simulink model "Lab3_HallLog_hw"  (R2025b)
settings: Solver=FixedStepDiscrete  StartTime=0.0  StopTime=inf  FixedStep=50e-6  RelTol=1e-3  EnableMultiTasking=on
undefined symbols (not defined in the file or in its folder): A0, A4, ADC, B0, C10, C11, C12, C13, C14, C15, C2, C3, C4, C5, D0, D1, D10, D12, D13, D14, D2, D3, D5, D6, D9, DiscIntNeverNeededParam, Max, MaxPer, ms, NumBits1, NumBits2, P1, P17, P20, P35, P36, P37, P38, P43, P44, P45, P46, P47, P48, P49, P50, P51, P52, P54, P55, P58, P59, P61, P62, P63, Pin, PWM1_Trg1, Resol, s, us
libraries: simulink x29, MCHP_Blockset x18
(part 2 of 4)

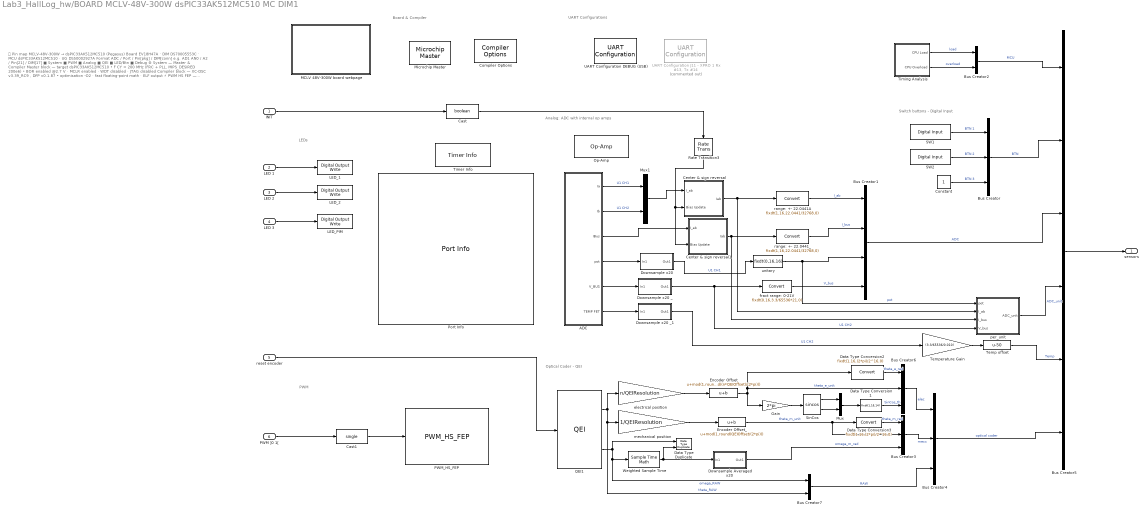
== system Lab3_HallLog_hw/BOARD MCLV-48V-300W dsPIC33AK512MC510 MC DIM1 ==
  note: Switch buttons - Digital Input
  note: LEDs
  note: UART Configurations
  note: PWM
  note: Optical Coder - QEI
  note: Analog: ADC with internal op amps
  note: Board & Compiler
  note: 🔌 Pin map MCLV-48V-300W → dsPIC33AK512MC510 (Pegasus)
      | Board EV18H47A · DIM DS70005553C · MCU dsPIC33AK512MC510 · UG DS50002927A
      | Format ADC / Port / Pin[pkg] / DIM[conn] e.g. AD1 AN0 / A2 / Pin[21] / DIM[17]
      | ■ System ■ PWM ■ Analog ■ QEI ■ LED/Btn ■ Debug
      | ⚙ System — Master & Compiler
      | Master block — target dsPIC33AK512MC510
      | • F CY = 200 MHz (FRC + PLL, MIPS_DESIRED 200e6)
      | • BOR enabled @2.7 V · MCLR enabled · WDT disabled · JTAG disabled
      | Compiler block — XC-DSC v3.39_RC9 , DFP v0.1.87
      | • optimisation -O2 · fast floating-point math · ELF output
      | ⚡ PWM HS FEP — 3-phase motor drive
      | PWM_HS_FEP — center-aligned, complementary (H/L pairs):
      | • period 50 µs = 20 kHz · dead-time 2 µs · resolution 0.275 µs
      | • PG1 triggers ADC (conversion synced to PWM) · channels 1-3 used
      | RD2 / Pin[82] / DIM[ 1] M1_PWM_AH RD3 / Pin[83] / DIM[ 3] M1_PWM_AL
      | RD0 / Pin[78] / DIM[ 5] M1_PWM_BH RD1 / Pin[79] / DIM[ 7] M1_PWM_BL
      | RC3 / Pin[66] / DIM[ 2] M1_PWM_CH RC4 / Pin[67] / DIM[ 4] M1_PWM_CL
      | 🌙 Analog — current & voltage sense
      | Phase & bus current — internal Op-Amp path (on-chip OA1/OA2/OA3 of the Pegasus DIM):
      | • R sh = 0.003 Ω × A v,DIM = 25 ⇒ 75 mV/A, biased at 1.65 V (V ref = Avdd/2)
      | • full scale = ±22.0441 A (firmware 22.0441/2^15 ) (DIM DS70005553C )
      | • External Op-Amp alt. : baseboard shunt 0.01 Ω + baseboard amp; jumpers DS50002927A Table 3-2
      | DC-bus voltage — resistor divider ( DS50002927A §3.2.5, Fig. 3-5) :
      | • R87/(R69+R77+R87) = 3.3/(34+34+3.3) = 1/21.6 ⇒ V bus,fs ≈ 69–71 V (firmware 3.3/2^16×21 )
      | AD1 AN0 / A2 / Pin[21] / DIM[17] M1_IA (OA1OUT)
      | AD2 AN0 / B0 / Pin[31] / DIM[25] M1_IB (OA2OUT)
      | AD3 AN0 / A5 / Pin[24] / DIM[33] M1_IBUS (OA3OUT)
      | A4 / Pin[23] OA1 IN+ A3 / Pin[22] OA1 IN-
      | B2 / Pin[33] OA2 IN+ B1 / Pin[32] OA2 IN-
      | B5 / Pin[26] OA3 IN+ A6 / Pin[25] OA3 IN-
      | ⚙ QEI · 💡 Digital I/O (LEDs & buttons)
      | LEDs = Digital Outputs · SW1/SW2 = Digital Inputs · QEI = quadrature encoder A/B.
      | RD14 / Pin[96] / DIM[42] M1_QEI_A RE2 / Pin[10] / DIM[30] M1_LED1 (DOut)
      | RD13 / Pin[95] / DIM[44] M1_QEI_B RE3 / Pin[ 6] / DIM[32] M1_LED2 (DOut)
      | RF1 / Pin[38] LED_DIM (DOut)
      | RA12 / Pin[ 3] / DIM[34] SW1 (M1_BUTTON1) (DIn)
      | RE1 / Pin[ 2] / DIM[36] SW2 (M1_BUTTON2) (DIn)
      | 🖥 Debug UART / programming
      | UART1 (DEBUG / USB) — 460800 baud , 8-N-1, Tx via DMA circular buffer.
      | Reaches the PC over the on-board USB-UART bridge → USB CDC virtual COM port
      | ( DS50002927A §2.2.3, J6) .
      | RC15 / Pin[75] / DIM[52] DEBUG_TX (U1TX)
      | RC14 / Pin[74] / DIM[54] DEBUG_RX (U1RX)
      | 🔗 Product page · Board User's Guide · DIM info sheet
  INIT : Inport
  LED 1 : Inport  Port=2
  LED 2 : Inport  Port=3
  LED 3 : Inport  Port=4
  reset encoder : Inport  Port=5
  PWM ]0 1[ : Inport  Port=6  Unit=1
  ADC : Subsystem
  Bus Creator{,3..4,6} (4 alike) : BusCreator  Inputs=3
  Bus Creator1 : BusCreator  Inputs=4
  Bus Creator2 : BusCreator  Inputs=2
  Bus Creator5 : BusCreator  Inputs=6
  Bus Creator7 : BusCreator  Inputs=2
  Cast : DataTypeConversion  OutDataTypeStr=boolean  SaturateOnIntegerOverflow=off  RndMeth=Floor
  Cast1 : DataTypeConversion  OutDataTypeStr=single  SaturateOnIntegerOverflow=off  RndMeth=Floor
  Center & sign reversal : Subsystem
  Center & sign reversal1 : Subsystem
  Compiler Options : MCHP_Blockset/System Configuration/Compiler Options  Priority=1  LATEST_CMPLR=on  COMP_LIST_TXT=XC-DSC - v4.00  DFP_LIST_TXT=v 1.4.172  CMSIS_DSP_TXT=Dynamic Options  USE_64BIT_DOUBLE=off  MCHP_MULTITHREAD_COMPILATION=on  UseCustom_LinkerScript=off  MCHP_MASTERLINK=Lab3_HallLog_hw_solution/BOARD MCLV-48V-300W dsPIC33AK512MC510 MC DIM1/Microchip Master  OPTIMIZATION_LEVEL=2  MPLAB_LINKLIB=default  MPLAB_LINKLIB1=fast floating-point math  CodeReplacement_TXT=None  OPTIMIZATION_FLTO=off  OPTIMIZATION_REORDER=off  OPTIMIZATION_ASM_REORDER=on  UNROLL_LOOPS=off  PROCEDURAL_ABSTRACTION=off  CONSERVE_STACK=off  GC_SECTIONS=None  MCODE=is more than 32768  MCONST=in data memory  MDATA=Can use all available memory  MSCALAR=Can use all available memory  MLARGEARRAY=off  MAGGREGATE=off  HEAP_SIZE=1024  OMF=elf  DEBUG_INFO=on  MCHP_STACK_USAGE=off  GCC_STACK_USAGE=off  ProduceHexOutput=off  AssemblyListing=off  SaveTemps=off  NO_EDS_WARN=on  PRINT_STATISTICS=off
      settings: SourceProductName=MPLAB Device Blocks for Simulink
  Constant : Constant  OutDataTypeStr=boolean  SampleTime=-1
  Data Type Duplicate : DataTypeDuplicate
  Data Type Conversion1 : DataTypeConversion  OutDataTypeStr=fixdt(1,16,14)  RndMeth=Floor
  Data Type Conversion2 : DataTypeConversion  OutDataTypeStr=fixdt(1,16,(2*pi)/2^16,0)  ConvertRealWorld=Stored Integer (SI)  SaturateOnIntegerOverflow=off  RndMeth=Floor
  Data Type Conversion3 : DataTypeConversion  OutDataTypeStr=fixdt(1,16,(2*pi)/2^16,0)  ConvertRealWorld=Stored Integer (SI)  SaturateOnIntegerOverflow=off  RndMeth=Floor
  Downsample Averaged x20 : Subsystem  mask{DownSample=10}
      mask prompts: DownSample "DownSample Factor"
  Downsample x20 : Subsystem  mask{DownSample=20}
      mask prompts: DownSample "DownSample Factor"
  Downsample x20 _ : Subsystem  mask{DownSample=20}
      mask prompts: DownSample "DownSample Factor"
  Downsample x20 _1 : Subsystem  mask{DownSample=20}
      mask prompts: DownSample "DownSample Factor"
  Encoder Offset : Bias  Bias=mod(1,round((n*QEIOffset)/(2*pi)))  SaturateOnIntegerOverflow=off
  Encoder Offset_ : Bias  Bias=mod(1,round(QEIOffset/(2*pi)))  SaturateOnIntegerOverflow=off
  Gain : Gain  Gain=2*pi  ParamDataTypeStr=single  OutDataTypeStr=single
  LED_1 : MCHP_Blockset/Digital IO/Digital Output Write  PORT_TXT="E   [ 0 : 4 ]"  PIN=2  INIT_VALUE=-1  PACK=off  OUTPUT_PIN_MODE=Push-Pull (default)  SIMULTANEOUS=off  ORDERING=None  SampleTime=-1  MCHP_PORT={Digital Out}{DOU}1:1:E2;  MCHP_MASTERLINK=Lab3_HallLog_hw_solution/BOARD MCLV-48V-300W dsPIC33AK512MC510 MC DIM1/Microchip Master
      settings: SourceProductName=MPLAB Device Blocks for Simulink
  LED_2 : MCHP_Blockset/Digital IO/Digital Output Write  PORT_TXT="E   [ 0 : 4 ]"  PIN=3  INIT_VALUE=-1  PACK=off  OUTPUT_PIN_MODE=Push-Pull (default)  SIMULTANEOUS=off  ORDERING=None  SampleTime=-1  MCHP_PORT={Digital Out}{DOU}1:1:E3;  MCHP_MASTERLINK=Lab3_HallLog_hw_solution/BOARD MCLV-48V-300W dsPIC33AK512MC510 MC DIM1/Microchip Master
      settings: SourceProductName=MPLAB Device Blocks for Simulink
  LED_PIM : MCHP_Blockset/Digital IO/Digital Output Write  PORT_TXT="F   [ 0 : 3 ]"  PIN=1  INIT_VALUE=-1  PACK=off  OUTPUT_PIN_MODE=Push-Pull (default)  SIMULTANEOUS=off  ORDERING=None  SampleTime=-1  MCHP_PORT={Digital Out}{DOU}1:1:F1;  MCHP_MASTERLINK=Lab3_HallLog_hw_solution/BOARD MCLV-48V-300W dsPIC33AK512MC510 MC DIM1/Microchip Master
      settings: SourceProductName=MPLAB Device Blocks for Simulink
  MCLV 48V-300W board webpage : Subsystem
      settings: OpenFcn=|
      | web('https://www.microchip.com/en-us/development-tool/EV62P66A','-browser'); % dsPIC33CK256MP508 DIM
      | pause(1);
      | web('https://www.microchip.com/en-us/development-tool/EV18H47A','-browser'); % LVMC 300W
      mask Display: image('MCHP_i_Board_MCLV_300W48V_reduced.jpg');
  Microchip Master : MCHP_Blockset/System Configuration/Microchip Master  Priority=1  PICREF=33AK512MC510  TIMESTEP_REF=PWM1_Trg1 + ADC  BUSYFLAG_TXT=None  PWRTEN=Not used  BOREN=Enabled  BODENV=2.7V  BORV=Not used  FPWRT=64ms  DSBOREN=Enable ZPBOR during Deep Sleep Mode  DSLPBOR=Not used  MCLRE=Enabled  SMCLR=MCLR pin generates a normal system Reset  PMDL1WAY=Allow only one reconfiguration  RSTPRI=Device will obtain reset instruction from Primary flash  TEMP=Not used  SOSCSRC=Not used  SOSCSEL=Not used  IOL1WAY=Allow only one reconfiguration  ALTVREF=Not used  DISUVREG=Not used  DSSWEN=Not used  LPCFG=Not used  RTCBAT=Not used  VBTBOR=Not used  WUTSEL=Not used  POWERSAVE=off  FNOSC=Internal Fast RC (FRC)  FPR=ECIO w/ PLL 16x  FOSFPR=Internal Fast RC (No change to Primary Osc Mode bits)  FOS=Primary Oscillator  FRANGE=High Range  OSCILLATOR_SELECT=External Clock  OSCILLATOR_SELECT_spd=External Clock  QUARTZ=8e6  QUARTZ_spd=8e6  FRC_TUNE_Range12_Step0P375=0.000 %  FRC_TUNE_Range12_Step0P375_CUSTOM=0  FRC_TUNE_Range1P5_Step0P047=0.000 %  FRC_TUNE_Range1P5_Step0P047_CUSTOM=0  BFRC_TUNE_Range1P5_Step0P047=0.000 %  BFRC_TUNE_Range1P5_Step0P047_CUSTOM=0  POSCGAIN=2x gain setting  POSCBOOST=Boost the kick start of the oscillator  SOSCGAIN=2x gain setting  SOSCBOOST=Boost the kick start of the oscillator  ACTIV_PLL=on  ACTIV_PLL_spd=on  MIPS_DESIRED=200e6  MIPS_DESIRED_spd=200e6  CPUDIV=Divide by 1  FPLLMUL=Not used  FPLLIDIV=8x Divider  POSCFREQ=Not used  POSCMD=Primary Oscillator Disabled  POSCMOD=Primary osc disabled  MIPS=200 * 1e6  ACLKCON=Optimized for PWM resolution & ADC conversion speed  ACLKCON_spd=Optimized for PWM resolution & ADC conversion speed  FPLLODIV=32x Divider  PLLKEN=Clock switch to PLL source will wait until the PLL lock signal is valid  FCKSM=Both Clock switching and Fail-safe Clock Monitor are disabled  FCKSMEN=Sw Disabled; Mon Disabled  IESO=Start up with FRC; then switch  DSWDTPS=1:2^36  FWDTEN=Disable  FWDTWINSZ=Window size is 25%  FWPSA=1:512  FWPSA0=1:128  FWPSB=1:16  WDT=Disable  WDTPOST=1:32768  WDTPRE=1:128  WDTPS=1:1048576  WINDIS=Watchdog Timer operates in Non-Window mode  WWDTEN=Non-Window mode  DSWDTEN=Enable DSWDT during Deep Sleep Mode  DSWDTOSC=Select LPRC as DSWDT Reference clock  FWDT_RCLKSEL=WDT Run Mode uses 32.78kHz clock from BFRC/244  FWDT_RWDTPS=1:2147483648  FWDT_SWDTMPS=1:2147483648  FWDT_WDTEN=WDT is controlled by software; use WDTCON.ON bit  FWDT_WDTRSTEN=WDT event generates a reset  FWDT_WDTWIN=WDT Window is 25% of WDT period  FWDT_WINEN=Not used  FPBDIV=Not used  FSOSCEN=Disable Secondary Oscillator  LPRCSEL=Not used  OSCIOFCN=Not used  OSCIOFNC=general purpose digital I/O pin  LVRCFG=Not used  PLL_96MHZ=Not used  PLL96MHZ=Not used  PLLDIV=Not used  WDTCLK=Not used  WDTCMX=Not used  WDTWIN=WDT Window is 25% of WDT period  XTCFG=24-32 MHz crystals  XTBST=Boost the kick-start  APL=Aux Flash Code protect is disabled  APLK=Aux Flash Write Protection or Code Protection is Enabled  AWRP=Auxiliary program memory is not write-protected  BSS=No Boot Segment  BWP=Not used  BWRP=Boot Segment Program Memory may be written  CP=Protection Disabled  EBS=No Boot EEPROM  ESS=No Segment Data EEPROM  GCP=Disable  GSS=General Segment Code protect is Disabled  GSS0=Not used  GSSK=General Segment Write Protection or Code Protection is Enabled  GWRP=Disable  PWP=Not used  RBS=No Boot RAM  RSS=No Secure RAM  SSS=No Secure Segment  SWRP=Disable  WPCFG=Not used  WPDIS=Not used  WPEND=Not used  WPFP=Not used  ICESEL=Communicate on PGEC1/PGED1  ICS=Use PGC/EMUC and PGD/EMUD  JTAGEN=Disable  FICD_JTAGEN=Disable  COE=Not used  RES=Not used  DEBUG=Debugger is disabled  BACKBUG=Not used  BKBUG=Not used  ALTI2C=I2C mapped to SDA1/SCL1 pins  ALTI2C1=I2C1 mapped to SDA1/SCL1 pins  ALTI2C2=I2C2 mapped to SDA2/SCL2 pins  ALTI2C3=I2C3 mapped to SDA3/SCL3 pins  FDEVOPT1_ALTI2C1=Not used  FDEVOPT1_ALTI2C2=Not used  FDEVOPT1_SPI2MAPDIS=Not used  FDEVOPT_ALTI2C1=Primary I2C1 pins are used  FDEVOPT_ALTI2C2=Primary I2C2 pins are used  FDEVOPT_ALTI2C3=Primary I2C3 pins are used  FDEVOPT_SPI2PIN=SPI2 pins are selected by peripheral pin selection feature  ALTQIO=QEA1; QEB1; INDX1 are selected as inputs to QEI1  ALTSS1=SS1A is selected as the I/O pin for SPI1  CMPPOL0=Hysteresis is applied to falling edge  CMPPOL1=Hysteresis is applied to falling edge  FCANIO=Not used  FETHIO=Default Ethernet I/O  FMIIEN=MII Enabled  FSRSSEL=Not used  FUSBIDIO=Controlled by the USB Module  FVBUSONIO=Not used  HPOL=Active High  HYST0=45 mV Hysteresis  HYST1=45 mV Hysteresis  I2C1SEL=Not used  LPOL=Active High  PWMPIN=Control with PORT/TRIS regs  RTCOSC=Not used  UPLLEN=USB PLL Disabled  UPLLIDIV=Not used  ATMOD8=Not used  ALTPMP=Not used  I2C2SEL=Not used  ALTADREF=Not used  ALTCVREF=Not used  PWMLOCK=PWM registers may be written without key sequence  INT_PRIORITY_DMA=0  MCHP_TIMER_RESULT=[ ]  MCHP_PLLRegisters="[0        -1     16386        -1  16815713]"  MCHPVAR=MCHP.fcy.MIPS=2e+08;MCHP.fcy.SYSCLK=2e+08;MCHP.fcy.Fplli=8000000;MCHP.fcy.Fvco=1.2e+09;MCHP.fcy.Fpllo=2e+08;MCHP.fcy.PWM=2e+08;MCHP.fcy.ADC=80000000;MCHP.fcy.PDM_DAC=2e+08;MCHP.fcy.UART=2e+08;MCHP.fcy.SPI=2e+08;MCHP.fcy.BiSS=2e+08;MCHP.fcy.SCC=2e+08;MCHP.fcy.Timers=1e+08;MCHP.fcy.I2C=2e+08;MCHP.PowerSave=0;MCHP.TimeStepFactor=-20000;MCHP.TimeStep_Timer=-1;MCHP.NTIMERS=3;MCHP.id.name='33AK512MC510';MCHP.id.N=reshape([33 512 510],1,3);MCHP.id.L=reshape({ 'AK','MC',''},1,3);MCHP.id.Arch=8;MCHP.id.maskset='STX32_Pegasus';MCHP.id.masksetFamily='STX32_Pegasus';MCHP.id.dos='05308';MCHP.id.ds='70005591';MCHP.id.archTxt='33Axxx';MCHP.id.clonedfrom='DSPIC33AK128MC106';MCHP.id.isSlave=0;MCHP.id.isMaster=0;MCHP.periph.PPS.reg_RPINRx=reshape([-1 1 1 1 1 1 1 1 1 1 1 1 1 1 1 1 1 1 1 1 1 1 1 1 1 1 -1 -1 -1 -1 -1 -1 1 1 1 1 1 1 1 1 1 1 1 1 1 1 1 1 1 1 1 1 1 1 1 1 1 1 1 1 1 1 1 1 1 1 1 1 1 1 1 1 1 1 1 1 1 1 1 1 1 1 1 -1 -1 -1 -1 -1 -1 -1 -1 -1 -1 1 1 1 1 1 1 1 1 1 1 1 1 1 1 1 1 1 1],1,111);MCHP.periph.pin.ODCx=reshape([65535 65535 65535 65535 31 15 7 0 0 0 0],1,11);MCHP.PPS.dsPIC.RP=reshape([-1 0 1 2 3 4 5 6 7 8 9 10 11 12 13 14 15 16 17 18 19 20 21 22 23 24 25 26 27 28 29 30 31 32 33 34 35 36 37 38 39 40 41 42 43 44 45 46 47 48 49 50 51 52 53 54 55 56 57 58 59 60 61 62 63 64 65 66 67 68 -1 -1 -1 -1 -1 -1 -1 -1 -1 -1 -1 80 81 82 83 -1 -1 -1 -1 -1 -1 -1 -1 -1 -1 -1 -1 96 97 98],1,100);MCHP.PPS.dsPIC.RPI=[];MCHP.PPS.dsPIC.RPINR_list=reshape({ '1','INT1','INT2','INT3','INT4','T1CK','T2CK','T3CK','TCKI1','ICM1','TCKI2','ICM2','TCKI3','ICM3','TCKI4','ICM4','TCKI5','ICM5','TCKI6','ICM6','TCKI7','ICM7','TCKI8','ICM8','TCKI9','ICM9','27','28','OCFA','OCFB','OCFC','OCFD','PCI8','PCI9','PCI10','PCI11','QEIA1','QEIB1','QEINDX1','QEIHOM1','QEIA2','QEIB2','QEINDX2','QEIHOM2','QEIA3','QEIB3','QEINDX3','QEIHOM3','QEIA4','QEIB4','QEINDX4','QEIHOM4','U1RX','U1DSR','U2RX','U2DSR','U3RX','U3DSR','SDI1','SCK1_in','SS1_in','SDI2','SCK2_in','SS2_in','SDI3','SCK3_in','SS3_in','SDI4','SCK4_in','SS4_in','C1RX','C2RX','SENT1','SENT2','REFI1','REFI2','PCI12','PCI13','PCI14','PCI15','PCI16','PCI17','PCI18','CLCINA','CLCINB','CLCINC','CLCIND','CLCINE','CLCINF','CLCING','CLCINH','CLCINI','CLCINJ','ADTRG31','U1CTS','U2CTS','U3CTS','BISSSL1','BISSGS1','IOMON1F12','IOMON1F13','IOMON1F14','IOMON1F15','IOMON2F12','IOMON2F13','IOMON2F14','IOMON2F15','PCI19','PCI20','PCI21','PCI22'},1,111);MCHP.PPS.dsPIC.RPOR_list=reshape({ '1','PWM1H','PWM1L','PWM2H','PWM2L','PWM3H','PWM3L','PWM4H','PWM4L','PWM5H','PWM5L','PWM6H','PWM6L','PWM7H','PWM7L','PWM8H','PWM8L','CAN1TX','CAN2TX','U1TX','U1RTS','U2TX','U2RTS','U3TX','U3RTS','SDO1','SCK1_out','SS1_out','SDO2','SCK2_out','SS2_out','SDO3','SCK3_out','SS3_out','SDO4','SCK4_out','SS4_out','REFO1','REFO2','OCM1','OCM2','OCM3','OCM4','OCM5','OCM6','OCM7','OCM8','MCCP_OCM1A','MCCP_OCM1B','MCCP_OCM1C','MCCP_OCM1D','MCCP_OCM1E','MCCP_OCM1F','CMPO1','CMPO2','CMPO3','CMPO4','CMPO5','CMPO6','CMPO7','CMPO8','PWME1','PWME2','PWME3','PWME4','QEICMP1','QEICMP2','QEICMP3','QEICMP4','CLC1OUT','CLC2OUT','CLC3OUT','CLC4OUT','CLC5OUT','CLC6OUT','CLC7OUT','CLC8OUT','CLC9OUT','CLC10OUT','PTGTRG24','PTGTRG25','SENT1OUT','SENT2OUT','BISSMO1','BISSMA1','U1DTR','U2DTR','U3DTR','APWM1H','APWM1L','APWM2H','APWM2L','APWM3H','APWM3L','APWM4H','APWM4L','APWME1','APWME2'},1,98);MCHP.PPS.dsPIC.RPV=reshape([-1 -1 -1 -1 -1 -1],1,6);MCHP.PPS.map_RPnR_RPORx=reshape([1 2 3 4 5 6 7 8 9 10 11 12 13 14 15 16 17 18 19 20 21 22 23 24 25 26 27 28 29 30 31 32 33 34 35 36 37 38 39 40 41 42 43 44 45 46 47 48 49 50 51 52 53 54 55 56 57 58 59 60 61 62 63 64 65 66 67 68 69 -1 -1 -1 -1 -1 -1 -1 -1 -1 -1 -1 81 82 83 84 -1 -1 -1 -1 -1 -1 -1 -1 -1 -1 -1 -1 97 98 99 -1 -1 -1 -1 -1 -1 -1 107 -1 -1 -1 -1 -1 -1 -1 -1 -1 -1 -1 -1 -1 -1 -1 -1 -1 -1 -1 -1 -1 129 130 131 132 133 134 135 136 137 138 139 140 141 142 143 144],1,144);MCHP.Rx=reshape([4 31 62 78 1 37 51 -1 -1 -1 -1 7 32 63 79 2 38 52 -1 -1 -1 -1 21 33 64 82 10 39 53 -1 -1 -1 -1 22 43 66 83 6 49 -1 -1 -1 -1 -1 23 44 67 92 16 -1 -1 -1 -1 -1 -1 24 26 65 90 -1 -1 -1 -1 -1 -1 -1 25 45 58 91 -1 -1 -1 -1 -1 -1 -1 5 46 59 98 -1 -1 -1 -1 -1 -1 -1 13 34 56 99 -1 -1 -1 -1 -1 -1 -1 14 35 57 76 -1 -1 -1 -1 -1 -1 -1 15 47 68 77 -1 -1 -1 -1 -1 -1 -1 12 48 69 93 -1 -1 -1 -1 -1 -1 -1 3 27 70 94 -1 -1 -1 -1 -1 -1 -1 11 30 71 95 -1 -1 -1 -1 -1 -1 -1 20 42 74 96 -1 -1 -1 -1 -1 -1 -1 17 36 75 97 -1 -1 -1 -1 -1 -1 -1],11,16);MCHP.ADC.ANtype=reshape([3 1],1,2);MCHP.ADC.ADCONx=reshape([4294804960 0 0 0 0 0],1,6);MCHP.ADC.ADCHS_0=reshape([0 0],1,2);MCHP.ADC.Flags=reshape([1 0],1,2);MCHP.ADC.Buffer=reshape([-1 -1],1,2);MCHP.ADC.port=reshape([-1 -1 -1 -1 -1 -1 -1 -1 -1 -1 -1 -1 -1 -1 -1 -1 -1 -1 -1 -1 -1 -1 -1 -1 -1 -1 -1 -1 -1 -1 -1 -1 -1 -1 -1 -1 -1 -1 -1 -1 -1 -1 -1 -1 -1 -1 -1 -1 -1 -1 -1 -1 -1 -1 -1 -1 -1],1,57);MCHP.ADC.port_ALT=reshape([-1 -1 -1 -1],1,4);MCHP.ADC.port_ALTA=reshape([-1 -1 -1 -1],1,4);MCHP.ADC.port_ALTB=reshape([-1 -1 -1 -1],1,4);MCHP.ADC.port_ALTC=reshape([-1 -1 -1 -1],1,4);MCHP.ADC.port_VrefP=-1;MCHP.ADC.port_VrefM=-1;MCHP.ADC.port_AVdd=-1;MCHP.ADC.port_AVss=-1;MCHP.ADC.ADCDATA=reshape([0 0 0 0 0 0 0 0 0 0 0 0 0 0 0 0 0 0 0 0 0 0 0 0 0 0 0 0 0 0 0 0 0 0 0 0 0 0 0 0 0 0 0 0 0 0 0 0 0 0 0 0 0 0 0 0 0],1,57);MCHP.ADC.HS_SAR.TRGSRC=reshape([0 0 0 0 0 0 0 0 0 0 0 0 0 0 0 0 0 0 0 0 0 0 0 0 0 0 0 0 0 0 0 0],1,32);MCHP.ADC.HS_SAR.nFilters=0;MCHP.ADC.HS_SAR.nDedicatedCore=0;MCHP.ADC.HS_SAR.CALIBRATION=0;MCHP.ADC.HS_SAR.ADCON1L=-1;MCHP.ADC.HS_SAR.ADC_Class3_idxStart=32;MCHP.memory.RAM=32768;MCHP.memory.RAM_XBegin=16384;MCHP.memory.RAM_YBegin=49152;MCHP.memory.RAM_dma=reshape([-1 -1],1,2);MCHP.memory.FLASH_ECC=0;MCHP.DMA.Num=8;MCHP.DMA.CNTmax=MCHP_Fun.Hex2num('41EFFFFFFFE00000');MCHP.QEI.QEICONx=reshape([49023 49023 49023 49023 -1 -1],1,6);MCHP.QEI.QEItype=4;MCHP.QEI.Port_QEI_INDX=reshape([-1 -1],1,2);MCHP.QEI.Port_QEI_QEA=reshape([-1 -1],1,2);MCHP.QEI.Port_QEI_QEB=reshape([-1 -1],1,2);MCHP.QEI.Port_QEI_UPDN=reshape([-1 -1],1,2);MCHP.INT.Port=reshape([5 32767 32767 32767 32767],1,5);MCHP.ADC1.port=reshape([2 4 3 9 10 -1 -1 -1 -1 -1 -1 -1 -1 -1 -1 -1 -1 -1 -1 -1 -1 -1 -1 -1 -1 -1 -1 -1 -1 -1 -1 -1],1,32);MCHP.ADC2.port=reshape([16 18 17 25 24 31 -1 -1 -1 -1 -1 -1 -1 -1 -1 -1 -1 -1 -1 -1 -1 -1 -1 -1 -1 -1 -1 -1 -1 -1 -1 -1],1,32);MCHP.ADC3.port=reshape([5 21 6 29 80 0 -1 -1 -1 -1 -1 -1 -1 -1 -1 -1],1,16);MCHP.ADC4.port=reshape([20 22 23 19 26 21 -1 -1 -1 -1 -1 -1 -1 -1 -1 -1],1,16);MCHP.ADC5.port=reshape([7 1 11 8 4 -1 -1 -1 -1 -1 -1 -1 -1 -1 -1 -1],1,16);MCHP.ADC1N.port=reshape([-1 10 3 -1 -1 -1 -1 -1 -1 -1],1,10);MCHP.ADC2N.port=reshape([-1 25 17 -1 -1 -1 -1 -1 -1 -1],1,10);MCHP.ADC3N.port=reshape([-1 29 6 -1],1,4);MCHP.ADC4N.port=reshape([-1 23 22 -1],1,4);MCHP.ADC5N.port=reshape([-1 7 11 -1],1,4);MCHP.PWM_HS.Flags=reshape([0 0 0],1,3);MCHP.PWM.port_FLT=reshape([-1 -1 -1 -1 -1 -1 -1 -1 -1 -1 -1 -1 -1 -1 -1 -1 -1 -1 -1 -1 -1 -1 -1 -1 -1 -1 -1 -1 -1 -1 -1 -1 -1],1,33);MCHP.PWM.PWMRef=-1;MCHP.PWM.Flag=0;MCHP.PWM.Port_PWM_l=reshape([51 40 49 63 36 47 37 98 54 -1 58 -1 43 -1 45 -1 -1 -1 -1 -1 -1 -1 -1 -1],2,12);MCHP.PWM.Port_PWM_h=reshape([50 59 48 62 35 46 34 97 53 -1 57 -1 42 -1 44 -1 -1 -1 -1 -1 -1 -1 -1 -1],2,12);MCHP.PWM_HS_FEP.nEVTOUT=5;MCHP.IC.Port=reshape([0 0 0 0 0 0 0 0 0 0 0 0 0 0 0 0],1,16);MCHP.IC.type=-1;MCHP.OC.Port=reshape([0 0 0 0 0 0 0 0 0 0 0 0 0 0 0 0],1,16);MCHP.OC.type=-1;MCHP.CN.Port=reshape([-1 -1 -1 -1 -1 -1 -1 -1 -1 -1 -1 -1 -1 -1 -1 -1 -1 -1 -1 -1 -1 -1 -1 -1 -1 -1 -1 -1 -1 -1 -1 -1 -1 -1 -1 -1 -1 -1 -1 -1 -1 -1 -1 -1 -1 -1 -1 -1 -1 -1 -1 -1 -1 -1 -1 -1 -1 -1 -1 -1 -1 -1 -1 -1 -1 -1 -1 -1 -1 -1 -1 -1 -1 -1 -1 -1 -1 -1 -1 -1 -1 -1 -1 -1 -1],1,85);MCHP.CN.PullUp=reshape([65535 65535 65535 65535 31 15 7 0 0 0 0],1,11);MCHP.CN.type=2;MCHP.CN.Flag_PullDown=1;MCHP.SPI.Refs=reshape([1 2 3 4 0 0],1,6);MCHP.SPI.SPIxCON1=-1;MCHP.SPI.SPIxCON2=-1;MCHP.SPI.SPIxFIFOSIZE=1;MCHP.SPI.Port_SDI=reshape([-1 27 -1 -1 -1 -1],1,6);MCHP.SPI.Port_SDO=reshape([-1 41 -1 -1 -1 -1],1,6);MCHP.SPI.Port_SCK=reshape([-1 26 -1 -1 -1 -1],1,6);MCHP.SPI.Port_SS=reshape([-1 -1 -1 -1 -1 -1],1,6);MCHP.I2C.Refs=reshape([1 2 3 0 0],1,5);MCHP.I2C.I2CxCON=58703615;MCHP.I2C.NewRegName=4;MCHP.I2C.Port_SDA=reshape([19 7 39 -1 -1],1,5);MCHP.I2C.Port_SCL=reshape([20 0 38 -1 -1],1,5);MCHP.I2C.Port_ASDA=reshape([54 56 60 -1 -1],1,5);MCHP.I2C.Port_ASCL=reshape([53 55 52 -1 -1],1,5);MCHP.I2C.Fuse_Port_SCL_SDA=reshape([9 1 10 1 11 1 -1 -1 -1 -1],2,5);MCHP.I2C.Fuse_Port_ASCL_ASDA=reshape([9 2 10 2 11 2 -1 -1 -1 -1],2,5);MCHP.SCCP.nSCCP=9;MCHP.SCCP.MCCP=reshape([1 1 1 1 1 1 1 1 1],1,9);MCHP.PGA.Port_PGA1P=reshape([-1 -1 -1 -1],1,4);MCHP.PGA.Port_PGA1N=reshape([-1 -1 -1 -1],1,4);MCHP.PGA.Port_PGA2P=reshape([-1 -1 -1 -1],1,4);MCHP.PGA.Port_PGA2N=reshape([-1 -1 -1 -1],1,4);MCHP.PGA.Num=0;MCHP.HS_AnalogComparator.Port_CMP1=reshape([2 4 3 14],1,4);MCHP.HS_AnalogComparator.Port_CMP2=reshape([16 18 17 24],1,4);MCHP.HS_AnalogComparator.Port_CMP3=reshape([5 21 6 28],1,4);MCHP.HS_AnalogComparator.Port_CMP4=reshape([19 20 23 1],1,4);MCHP.HS_AnalogComparator.Port_CMP5=reshape([8 9 10 13],1,4);MCHP.HS_AnalogComparator.Port_CMP6=reshape([0 7 11 -1],1,4);MCHP.HS_AnalogComparator.Port_CMP7=reshape([9 27 64 22],1,4);MCHP.HS_AnalogComparator.Port_CMP8=reshape([26 30 65 25],1,4);MCHP.HS_AnalogComparator.Port_CMPN=reshape([-1 -1 3 6 10 11],1,6);MCHP.HS_AnalogComparator.Port_EXTREFx=reshape([-1 -1],1,2);MCHP.HS_AnalogComparator.Port_DACOUTx=reshape([1 8],1,2);MCHP.HS_AnalogComparator.Num=4;MCHP.Comp.Port_CVrefin=-1;MCHP.Comp.Port_CVref=-1;MCHP.Comp.Port_CVref1O=-1;MCHP.Comp.Port_CVref2O=-1;MCHP.Comp.Port_CxOUT=reshape([32767 32767 32767 32767 32767],1,5);MCHP.Comp.Port_OAxOUT=reshape([2 16 5 -1 -1],1,5);MCHP.Comp.Port_CxINP=reshape([-1 -1 -1 -1 -1],1,5);MCHP.Comp.Port_CxINM=reshape([-1 -1 -1 -1 -1 -1 -1 -1 -1 -1 -1 -1 -1 -1 -1 -1 -1 -1 -1 -1],4,5);MCHP.Comp.Port_OAxINP=reshape([4 18 21 -1 -1],1,5);MCHP.Comp.Port_OAxINM=reshape([3 17 6 -1 -1],1,5);MCHP.Comp.nComp=reshape([5 0 0],1,3);MCHP.Comp.OpAmp=0;MCHP.Comp.CVRCON=reshape([0 0],1,2);MCHP.Comp.CMCON=0;MCHP.CDAC.Port_DACx=reshape([-1 -1 -1],1,3);MCHP.CDAC.nCDAC=4;MCHP.UART.port_Rx=reshape([32767 32767 32767 -1 -1 -1],1,6);MCHP.UART.port_Tx=reshape([32767 32767 32767 -1 -1 -1],1,6);MCHP.UART.port_ARx=reshape([-1 -1],1,2);MCHP.UART.port_ATx=reshape([-1 -1],1,2);MCHP.UART.port_RTS=reshape([32767 32767 32767 -1 -1 -1],1,6);MCHP.UART.port_CTS=reshape([32767 32767 32767 -1 -1 -1],1,6);MCHP.UART.reg_UxMODE=reshape(MCHP_Fun.Hex2num('[41E9FFF77FE00000 41E9FFF77FE00000 41E9FFF77FE00000 BFF0000000000000 BFF0000000000000 BFF0000000000000]'),1,6);MCHP.UART.reg_UxSTA=reshape(MCHP_Fun.Hex2num('[41DDFFFFFFC00000 41DDFFFFFFC00000 41DDFFFFFFC00000 BFF0000000000000 BFF0000000000000 BFF0000000000000]'),1,6);MCHP.modsrc.DOS_04094_cpu_33a_v1_dspic33a=1;MCHP.modsrc.DOS_04436_perseus_dspic33a=0;MCHP.modsrc.DOS_04928_gpio_ports_upb_v2_dspic33a=1;MCHP.modsrc.DOS_02672_math_progcrc_upb_v1_dspic33a=1;MCHP.modsrc.DOS_04993_sec_32bit_cp_upb_v1_dspic33a=1;MCHP.modsrc.DOS_03459_adc_pc_ctrl_upb_v2_dspic33a=0;MCHP.modsrc.DOS_04302_pwm_pc_upb_v3_dspic33a=0;MCHP.modsrc.DOS_03076_uart_protocol_upb_v1_dspic33a=1;MCHP.modsrc.DOS_01482_spi_i2s_upb_v1_dspic33a=1;MCHP.modsrc.DOS_05155_i2c_upb_v4_dspic33a=1;MCHP.modsrc.DOS_02359_sent_j2716_upb_v1_dspic33a=1;MCHP.modsrc.DOS_05177_qei_32b_upb_v2_dspic33a=1;MCHP.modsrc.DOS_01512_ccp_mccp_upb_v1_dspic33a=1;MCHP.modsrc.DOS_03496_dac_pdm_nbit_upb_v2_dspic33a=0;MCHP.modsrc.DOS_02673_tmr_classa_upb_v1_dspic33a=1;MCHP.modsrc.DOS_04776_perf_mon_upb_v1_dspic33a=1;MCHP.modsrc.DOS_03680_pfm_pbu_33a_upb_v1_dspic33a=1;MCHP.modsrc.DOS_04649_sec_pac_upb_v0_dspic33a=0;MCHP.modsrc.DOS_03966_io_integrity_monitor_upb_v1_dspic33a=1;MCHP.modsrc.DOS_04641_biss_master_upb_v1_dspic33a=1;MCHP.modsrc.DOS_04077_dma_upb_v1_dspic33a=1;MCHP.modsrc.DOS_04549_nvm_ctrl_32bit_upb_v1_dspic33a=1;MCHP.modsrc.DOS_04449_clk_cru_33a_upb_v1_dspic33a=1;MCHP.modsrc.DOS_03850_clk_monitor_upb_v1_dspic33a=1;MCHP.modsrc.DOS_04342_osc_rc8mhz_ctrl_upb_v4_dspic33a=1;MCHP.modsrc.DOS_04650_wdt_upb_v4_dspic33a=1;MCHP.modsrc.DOS_05178_ptg_pc_upb_v2_dspic33a=1;MCHP.modsrc.DOS_04181_data_ram_ctrl_upb_v1_dspic33a=1;MCHP.modsrc.DOS_04735_wdt_dmt_upb_v6_dspic33a=1;MCHP.modsrc.DOS_01577_cla_clc_upb_v1_dspic33a=1;MCHP.modsrc.DOS_03516_pwr_sib_upb_v3_dspic33a=0;MCHP.modsrc.DOS_03495_amp_pad_opamp_ctrl_upb_v2_dspic33a=1;MCHP.modsrc.DOS_02481_WACK_MC_Config=0;MCHP.modsrc.DOS_03088_pfm_cache_ocp_v2_WACK=0;MCHP.modsrc.DOS_02819_pfm_ctrl_32bit_upb_v2=0;MCHP.modsrc.DOS_02674_wdt_upb_v1_32bit=0;MCHP.modsrc.DOS_01520_wdt_dmt_upb_v1=0;MCHP.modsrc.DOS_02869_icd_jtag_bvci_upb_v2=0;MCHP.modsrc.DOS_02823_WACJ_clk_cru_upb_v2=0;MCHP.modsrc.DOS_02823_WACN_clk_cru_upb_v2=0;MCHP.modsrc.DOS_01423_RPINRx=0;MCHP.modsrc.DOS_02481_RPORx=0;MCHP.modsrc.DOS_02511_pwr_sib_upb_v1_32bit=0;MCHP.modsrc.DOS_02907_WACN_GP_int_evic_v3=0;MCHP.modsrc.DOS_01500_dma_bvci_v2=0;MCHP.modsrc.DOS_02141_tmr_classa_pb_v2=0;MCHP.modsrc.DOS_02815_tmr_classb_upb_v1=0;MCHP.modsrc.DOS_00740_icap_pb_v1=0;MCHP.modsrc.DOS_00749_ocmp_pb_v1=0;MCHP.modsrc.DOS_01441_i2c_upb_v1_32bit=0;MCHP.modsrc.DOS_01329_spi_pb_v2=0;MCHP.modsrc.DOS_02478_uart_irda_upb_v1_32bit=0;MCHP.modsrc.DOS_03554_cmp_control_upb_v2_32bit=0;MCHP.modsrc.DOS_01445_dac_nbit__control_upb_v1_32bit=0;MCHP.modsrc.DOS_01461_afe_ctmu_con_upb_v1=0;MCHP.modsrc.DOS_01577_cla_clc_upb_v1_32bit=0;MCHP.modsrc.DOS_02467_gpio_ports_upb_v1=0;MCHP.modsrc.DOS_02508_adc_sar_ctrl_upb_v1_PIC32MK=0;MCHP.modsrc.DOS_01261_tmr_rtcc_pb_v2=0;MCHP.modsrc.DOS_01475_lpwr_deep_sleep_ctrl_v2=0;MCHP.modsrc.DOS_EIP_00136_ssx_v1=0;MCHP.modsrc.DOS_02907_WACK_MC_int_evic_v3=0;MCHP.modsrc.DOS_02514_dfm_strl_sst_upb_v1=0;MCHP.modsrc.DOS_02472_ppi_pmp16_upb_v1=0;MCHP.modsrc.DOS_02813a_usb_otgcore_pb_v3=0;MCHP.modsrc.DOS_02481_WACP_Config=0;MCHP.modsrc.DOS_02907_WACP_int_evic_v3=0;MCHP.modsrc.DOS_01477_pwm_mc_upb_v1=0;MCHP.modsrc.DOS_01494_qei_32b_upb_v1=0;MCHP.modsrc.DOS_02508_WACP_adc_sar_ctrl_upb_v1=0;MCHP.modsrc.DOS_01261_tmr_rtcc_WACJ_K_N_P_pb_v2=0;MCHP.modsrc.DOS_02907_WACN_MC_int_evic_v3=0;MCHP.modsrc.DOS_03247_can_fd_upb_v2_pic32mk=0;MCHP.modsrc.DOS_02481_WACJ_MC_Config=0;MCHP.modsrc.DOS_02569_pfm_cache_ocp_v1=0;MCHP.modsrc.DOS_02481_WACJ_MC_int_evic_v3=0;MCHP.modsrc.DOS_01459_ptg_pc_upb_v1_SIC=0;MCHP.modsrc.DOS_01427_cmp_control_upb_v1_32bit=0;MCHP.modsrc.DOS_01152_can_bvci_v1=0;MCHP.modsrc.DOS_02787_WACD_Config=0;MCHP.modsrc.DOS_00800_dac_4bit_ctrl_pb_v1=0;MCHP.modsrc.DOS_01539_icd_jtag_pb_v2=0;MCHP.modsrc.DOS_02823_clk_cru_upb_v2=0;MCHP.modsrc.DOS_01423_RPORx=0;MCHP.modsrc.DOS_02907_WACD_int_evic_v3=0;MCHP.modsrc.DOS_00734_uart_irda_pb_v1=0;MCHP.modsrc.DOS_00687_tmr_classa_pb_v1=0;MCHP.modsrc.DOS_00745_tmr_classb_pb_v1=0;MCHP.modsrc.DOS_02508_adc_sar_ctrl_upb_v1=0;MCHP.modsrc.DOS_00866_cmp_control_pb_v2=0;MCHP.modsrc.DOS_01114_eth_bvci_v1=0;MCHP.modsrc.DOS_02831_usb_clk_rst_v2=0;MCHP.modsrc.DOS_01643_pfm_cache_ahb_v2=0;MCHP.modsrc.DOS_EIP_00206r5_sqi_v2=0;MCHP.modsrc.DOS_EIP_00124_usb_hs_otgcore_v1=0;MCHP.modsrc.DOS_EIP_00218_math_rng_ahbs_v2=0;MCHP.modsrc.DOS_EIP_00109_ebi_v1=0;MCHP.modsrc.DOS_EIP_00158_crypto_v1=0;MCHP.modsrc.DOS_05557_serpens_dspic33a=0;MCHP.modsrc.DOS_05972_adc_12b_upb_v3_adc_dspic33a=0;MCHP.modsrc.DOS_03681_bmx_33a_upb_v1_dspic33a=0;MCHP.modsrc.DOS_05226_pwm_pc_upb_v4_dspic33a=1;MCHP.modsrc.DOS_05514_qei_32b_upb_v3_dspic33a=0;MCHP.modsrc.DOS_02050_tmr_rtcc_upb_v1_dspic33a=0;MCHP.modsrc.DOS_05431_dac_pdm_nbit_upb_v3_dspic33a=1;MCHP.modsrc.DOS_04649_sec_pac_upb_serpens_dspic33a=0;MCHP.modsrc.DOS_05801_dma_upb_v2_dspic33a=0;MCHP.modsrc.DOS_05692_pwr_sib_upb_v5_dspic33a=0;MCHP.modsrc.DOS_05420_amp_vref_ctl_upb_v1_dspic33a=1;MCHP.modsrc.DOS_05346_sec_cam_v2_dspic33a=1;MCHP.modsrc.DOS_06006_adc_soft_code_seq_v2_adc_dspic33a=0;MCHP.modsrc.DOS_05442_icd_trace_33a_v1_dspic33a=0;MCHP.modsrc.DOS_04537_can_fd_upb_v3_dspic33a=1;MCHP.modsrc.DOS_05308_pegasus_dspic33a=1;MCHP.modsrc.DOS_02976_adc_12b_upb_v2_dspic33a=1;MCHP.modsrc.DOS_05404_adc_pc_ctrl_upb_v3_dspic33a=1;MCHP.modsrc.DOS_05226_apwm_pc_upb_v4_dspic33a=1;MCHP.modsrc.DOS_04649_sec_pac_upb_v1_dspic33a=1;MCHP.modsrc.DOS_05461_pwr_sib_upb_v4_dspic33a=1;MCHP.modsrc.DOS_03267_adc_soft_code_seq_v1_dspic33a=1;MCHP.modsrc.DOS_05830_blueRidge_dspic33a=0;MCHP.modsrc.DOS_05972_adc_12b_upb_v3_itc_dspic33a=0;MCHP.modsrc.DOS_05828_pfm_pbu_33a_upb_v2_dspic33a=0;MCHP.modsrc.DOS_05765_math_rdc_upb_v1_32bit=0;MCHP.modsrc.DOS_05908_math_cic_upb_v2_32bit=0;MCHP.modsrc.DOS_05592_pwr_monitor_sib_upb_v1=0;MCHP.modsrc.DOS_05924_bus_dual_die_upb_v2=0;MCHP.modsrc.DOS_06048_sec_cam_v3_dspic33a=0;MCHP.modsrc.DOS_05922_i3c_upb_v1_32bit=0;MCHP.modsrc.DOS_06006_adc_soft_code_seq_v2_dspic33a=0;MCHP.modsrc.DOS_02551_cpu_16bit_v7=0;MCHP.modsrc.DOS_01520_wdt_dmt_upb_v1_16bit=0;MCHP.modsrc.DOS_02359a_sent_j2716_upb_v1=0;MCHP.modsrc.DOS_02672_math_progcrc_upb_v1_16bit=0;MCHP.modsrc.DOS_01577_cla_clc_upb_v1=0;MCHP.modsrc.DOS_02915_ecc_v2=0;MCHP.modsrc.DOS_02673_tmr_classa_upb_v1_16bit=0;MCHP.modsrc.DOS_01494_qei_32b_upb_v1_16bit=0;MCHP.modsrc.DOS_01441_i2c_upb_v1_16bit_TLAH=0;MCHP.modsrc.DOS_03076_uart_protocol_upb_v1_16bit=0;MCHP.modsrc.DOS_01482=0;MCHP.modsrc.DOS_01483_pwm_16bit=0;MCHP.modsrc.DOS_04884_WAC0B=0;MCHP.modsrc.DOS_02316_nvm_ctrl_v1_16bit=0;MCHP.modsrc.DOS_03349_amp_pad_opamp_ctrl_upb_v1=0;MCHP.modsrc.DOS_02653_afe_current_bias_ctrl_upb_v1_16bit=0;MCHP.modsrc.DOS_01459_ptg_pc_upb_v1_16bit=0;MCHP.modsrc.DOS_01512_ccp_mccp_upb_v1_16bit=0;MCHP.modsrc.DOS_02519_dma_sfr_16bit_v2=0;MCHP.modsrc.DOS_02508c11=0;MCHP.modsrc.DOS_02475_dac_pdm_nbit_upb_v1_16bit=0;MCHP.modsrc.DOS_02467_gpio_upb_v1_16bit=0;MCHP.modsrc.DOS_00805_rst_integration_v4=0;MCHP.modsrc.DOS_02659_clk_sib_v12=0;MCHP.modsrc.DOS_02237_osc_dco_ctrl_upb_v1_16bit=0;MCHP.modsrc.DOS_02674_wdt_upb_v1_16bit=0;MCHP.modsrc.DOS_01407=0;MCHP.modsrc.DOS_03247_CAN_FD_UPB_V2_16_bit=0;MCHP.modsrc.DOS_03994_WAC07=0;MCHP.modsrc.DOS_02472_ppi_pmp16_upb_v1_16bit=0;MCHP.modsrc.DOS_02949_WACG=0;MCHP.modsrc.DOS_02552_msi_upb_v1_Master=0;MCHP.modsrc.DOS_03667_pwm_pc_upb_v2_16bit=0;MCHP.modsrc.DOS_04180_drm_ctrl_ecc_v1=0;MCHP.modsrc.DOS_03431_STX03=0;MCHP.modsrc.DOS_03516_pwr_sib_upb_v3=0;MCHP.modsrc.DOS_02552_msi_upb_v1_Slave=0;MCHP.modsrc.DOS_04621_amp_pga_ctrl_upb_v3=0;MCHP.modsrc.DOS_02497_WACV=0;MCHP.modsrc.DOS_02593_amp_pga_ctrl_pb_v2_16bit=0;MCHP.modsrc.DOS_03029_WACH=0;MCHP.modsrc.DOS_01483_apwm_16bit=0;MCHP.modsrc.DOS_04797_WAC0A=0;MCHP.modsrc.DOS_04797_WAC09=0;MCHP.modsrc.DOS_03662_WACU=0;MCHP.modsrc.DOS_00794=0;MCHP.modsrc.DOS_00931=0;MCHP.modsrc.DOS_00932=0;MCHP.modsrc.DOS_00942=0;MCHP.modsrc.DOS_00938=0;MCHP.modsrc.DOS_00996=0;MCHP.modsrc.DOS_00997=0;MCHP.modsrc.DOS_00998=0;MCHP.modsrc.DOS_00209=0;MCHP.modsrc.DOS_01555_adc=0;MCHP.modsrc.DOS_01293=0;MCHP.modsrc.DOS_00828=0;MCHP.modsrc.DOS_01116=0;MCHP.modsrc.DOS_01017_RPORx=0;MCHP.modsrc.DOS_01017_RPINRx=0;MCHP.modsrc.DOS_01555_nvm_tsmc18_v2_16bit=0;MCHP.modsrc.DOS_00804=0;MCHP.modsrc.DOS_00826=0;MCHP.modsrc.DOS_01555_TLAK_PMDx=0;MCHP.modsrc.DOS_01555_TLAK_INT_=0;MCHP.modsrc.DOS_00933=0;MCHP.modsrc.DOS_01555=0;MCHP.modsrc.DOS_01555_ptg=0;MCHP.modsrc.DOS_00929=0;MCHP.modsrc.DOS_00958=0;MCHP.modsrc.DOS_01117_PORTx=0;MCHP.modsrc.DOS_00999=0;MCHP.modsrc.DOS_01198=0;MCHP.modsrc.DOS_01041=0;MCHP.modsrc.DOS_00892=0;MCHP.modsrc.DOS_01287_TLAC_PMDx=0;MCHP.modsrc.DOS_01287_TLAC_INT_=0;MCHP.modsrc.DOS_01424=0;MCHP.modsrc.DOS_01332=0;MCHP.modsrc.DOS_01113=0;MCHP.modsrc.DOS_01017_PMDx=0;MCHP.modsrc.DOS_00927=0;MCHP.modsrc.DOS_01080=0;MCHP.modsrc.DOS_01468_PMBA_current_source=0;MCHP.modsrc.DOS_02291_PGA=0;MCHP.modsrc.DOS_01467_Comparator=0;MCHP.modsrc.DOS_01498_TLAY=0;MCHP.modsrc.DOS_00993_PLL_120MHz=0;MCHP.modsrc.DOS_01332_ptg_pc_v1=0;MCHP.modsrc.DOS_00958_pwm_TLAY=0;MCHP.modsrc.TLAY_IOPorts=0;MCHP.modsrc.DOS_00929q=0;MCHP.modsrc.DOS_02415_spi_v5=0;MCHP.modsrc.DOS_RPINRx_16bit_2=0;MCHP.modsrc.DOS_01497_TLAH_PMDx=0;MCHP.modsrc.DOS_02550_TLAL_INT=0;MCHP.modsrc.DOS_00958_pwm_TLAH=0;MCHP.modsrc.DOS_01287_TLAH_INT_=0;MCHP.modsrc.DOS_00794_cpu_16bit_v3=0;MCHP.modsrc.DOS_02192_TLCD_PMDx=0;MCHP.modsrc.DOS_02192_TLCD_INT_=0;MCHP.modsrc.DOS_02192_cmp=0;MCHP.modsrc.DOS_00958_pwm_TLCD=0;MCHP.modsrc.DOS_02192_PORTx_TLCD=0;MCHP.modsrc.DOS_00936=0;MCHP.modsrc.DOS_00995=0;MCHP.modsrc.DOS_00546=0;MCHP.modsrc.DOS_00474=0;MCHP.PortBase=16;MCHP.PortPrefixe='P';MCHP.clock.PBxDIV=-1;MCHP.clock.CLKx_INTDIV=reshape([-1 -1 -1 -1 0 1 0 0 0 -1 -1 0 0],1,13);MCHP.clock.CLKx_FRACDIV=reshape([-1 -1 -1 -1 0 256 0 0 0 -1 -1 0 0],1,13);MCHP.Scheduler.IE_ref=' ';MCHP.Scheduler.VectorName=' ';MCHP.Scheduler.IntPrefix=' ';MCHP.Scheduler.TimerIndex=-1;MCHP.Scheduler.Period_s=5e-05;MCHP.Scheduler.TIMESTEP_REF='PWM1_Trg1 + ADC';MCHP.Scheduler.TrigSourcePeriod_s=-1;  MCHP_CRC=19237870  BTMODE=Device is in Single Boot (legacy) mode  RES1=Not used  PLLSS=Not used  RES2=Not used  ALTCMPI=Not used  BOREN1=Not used  ALTRB6=Not used  RETCFG=Not used  DFMCY=Not used  BSS2=No Boot Segment  BSEN=No Boot Segment  CWRP=Configuration Segment may be written  CSS=No Protection (other than CWRP)  AIVTDIS=Disable Alternate Vector Table  BSLIM=Not used  AIVT_EN=off  BSLIM_EN=off  BSLIM_VAL=0x1FF0  WDTEN=Disable  BTSWP=BOOTSWP instruction is disabled  DBCC=No Cross Connection between DAC outputs  CTXT1=Not Assigned  CTXT2=Not Assigned  SEQNUM=Not used  nSEQNUM=Not used  BOREN0=Enabled  DMTIVT=Not used  DMTCNT=2^8 (256)  DMTEN=Dead Man Timer is Disabled and can be enabled by software  ON=Not used  USERID=Not used  RESERVED1=Not used  PGL1WAY=Allow only one reconfiguration  FPLLRNG=34-68 MHz Input  FPLLICLK=FRC is input to the System PLL  FPLLMULT=PLL Multiply by 128  UPLLFSEL=USB PLL input is 24 MHz  DMTINTV=Window/Interval value is 127/128 counter value  WDTSPGM=WDT stops during Flash programming  FDMTEN=Deadman Timer is disabled  TRCEN=Trace features in the CPU are enabled  BOOTISA=Boot code and Exception code is MIPS32  FECCCON=ECC and Dynamic ECC are disabled (ECCCON bits are writable)  EXTDDRSIZE=Not used  FSLEEP=Flash is powered down when the device is in Sleep mode  DBGPER=Allow CPU access to all permission regions  EJTAGBEN=Normal EJTAG functionality  TSEQ=Not used  CSEQ=Not used  RWDTPS=1:2147483648  RCLKSEL=Always use LPRC  SWDTPS=1:2147483648  DMTIVTL=Not used  DMTIVTH=Not used  DMTCNTL=Not used  DMTCNTH=Not used  DMTDIS=Dead Man Timer is Disabled and can be enabled by software  SMBEN=SMBus input threshold is enabled  SPI2PIN=SPI2 uses I/O remap (PPS) pins  CTXT3=Not Assigned  CTXT4=Not Assigned  MBXM0=Mailbox register configured for Main data read (Secondary to Main data transfer)  MBXM1=Mailbox register configured for Main data read (Secondary to Main data transfer)  MBXM2=Mailbox register configured for Main data read (Secondary to Main data transfer)  MBXM3=Mailbox register configured for Main data read (Secondary to Main data transfer)  MBXM4=Mailbox register configured for Main data read (Secondary to Main data transfer)  MBXM5=Mailbox register configured for Main data read (Secondary to Main data transfer)  MBXM6=Mailbox register configured for Main data read (Secondary to Main data transfer)  MBXM7=Mailbox register configured for Main data read (Secondary to Main data transfer)  MBXM8=Mailbox register configured for Main data read (Secondary to Main data transfer)  MBXM9=Mailbox register configured for Main data read (Secondary to Main data transfer)  MBXM10=Mailbox register configured for Main data read (Secondary to Main data transfer)  MBXM11=Mailbox register configured for Main data read (Secondary to Main data transfer)  MBXM12=Mailbox register configured for Main data read (Secondary to Main data transfer)  MBXM13=Mailbox register configured for Main data read (Secondary to Main data transfer)  MBXM14=Mailbox register configured for Main data read (Secondary to Main data transfer)  MBXM15=Mailbox register configured for Main data read (Secondary to Main data transfer)  MBXHSA=MSIxMBXD15 assigned to mailbox handshake protocol block A  MBXHSB=MSIxMBXD15 assigned to mailbox handshake protocol block B  MBXHSC=MSIxMBXD15 assigned to mailbox handshake protocol block C  MBXHSD=MSIxMBXD15 assigned to mailbox handshake protocol block D  MBXHSE=MSIxMBXD15 assigned to mailbox handshake protocol block E  MBXHSF=MSIxMBXD15 assigned to mailbox handshake protocol block F  MBXHSG=MSIxMBXD15 assigned to mailbox handshake protocol block G  MBXHSH=MSIxMBXD15 assigned to mailbox handshake protocol block H  HSAEN=Mailbox data flow control handshake protocol block disabled  HSBEN=Mailbox data flow control handshake protocol block disabled  HSCEN=Mailbox data flow control handshake protocol block disabled  HSDEN=Mailbox data flow control handshake protocol block disabled  HSEEN=Mailbox data flow control handshake protocol block disabled  HSFEN=Mailbox data flow control handshake protocol block disabled  HSGEN=Mailbox data flow control handshake protocol block disabled  HSHEN=Mailbox data flow control handshake protocol block disabled  CPRA0=Main core owns pin  CPRA1=Main core owns pin  CPRA2=Main core owns pin  CPRA3=Main core owns pin  CPRA4=Main core owns pin  CPRB0=Main core owns pin  CPRB1=Main core owns pin  CPRB2=Main core owns pin  CPRB3=Main core owns pin  CPRB4=Main core owns pin  CPRB5=Main core owns pin  CPRB6=Main core owns pin  CPRB7=Main core owns pin  CPRB8=Main core owns pin  CPRB9=Main core owns pin  CPRB10=Main core owns pin  CPRB11=Main core owns pin  CPRB12=Main core owns pin  CPRB13=Main core owns pin  CPRB14=Main core owns pin  CPRB15=Main core owns pin  CPRC0=Main core owns pin  CPRC1=Main core owns pin  CPRC2=Main core owns pin  CPRC3=Main core owns pin  CPRC4=Main core owns pin  CPRC5=Main core owns pin  CPRC6=Main core owns pin  CPRC7=Main core owns pin  CPRC8=Main core owns pin  CPRC9=Main core owns pin  CPRC10=Main core owns pin  CPRC11=Main core owns pin  CPRC12=Main core owns pin  CPRC13=Main core owns pin  CPRC14=Main core owns pin  CPRC15=Main core owns pin  CPRD0=Main core owns pin  CPRD1=Main core owns pin  CPRD2=Main core owns pin  CPRD3=Main core owns pin  CPRD4=Main core owns pin  CPRD5=Main core owns pin  CPRD6=Main core owns pin  CPRD7=Main core owns pin  CPRD8=Main core owns pin  CPRD9=Main core owns pin  CPRD10=Main core owns pin  CPRD11=Main core owns pin  CPRD12=Main core owns pin  CPRD13=Main core owns pin  CPRD14=Main core owns pin  CPRD15=Main core owns pin  CPRE0=Main core owns pin  CPRE1=Main core owns pin  CPRE2=Main core owns pin  CPRE3=Main core owns pin  CPRE4=Main core owns pin  CPRE5=Main core owns pin  CPRE6=Main core owns pin  CPRE7=Main core owns pin  CPRE8=Main core owns pin  CPRE9=Main core owns pin  CPRE10=Main core owns pin  CPRE11=Main core owns pin  CPRE12=Main core owns pin  CPRE13=Main core owns pin  CPRE14=Main core owns pin  CPRE15=Main core owns pin  S1FNOSC=Internal Fast RC (FRC) Oscillator with postscaler  S1IESO=Start up with FRC; then switch  S1OSCIOFNC=OSC2 is clock output  S1FCKSM=Both Clock switching and Fail-safe Clock Monitor are disabled  S1PLLKEN=S1PLLKEN_ON  S1RWDTPS=1:1048576  S1RCLKSEL=Always use LPRC  S1WINDIS=Watchdog Timer operates in Non-Window mode  S1WDTWIN=WDT Window is 25% of WDT period  S1SWDTPS=1:1048576  S1FWDTEN=use WDTCON.ON bit  S1ICS=Communicate on PGC1 and PGD1  S1DEBUG=Not used  S1ISOLAT=The Secondary can operate (in debug mode) even if the SLVEN bit in the MSI is zero  S1NOBTSWP=BOOTSWP instruction is disabled  S1ALTI2C1=I2C1 mapped to SDA1/SCL1 pins  S1SPI1PIN=Secondary SPI1 uses I/O remap (PPS) pins  S1SSRE=Secondary generated resets will reset the Secondary Enable Bit in the MSI module  S1MSRE=The Main software oriented RESET events (RESET Op-Code; Watchdog timeout; TRAP reset; illegalInstruction) will also cause the Secondary subsystem to reset  S1CTXT1=Not Assigned  S1CTXT2=Not Assigned  S1CTXT3=Not Assigned  S1CTXT4=Not Assigned  BORLVL=Not used  BSSO=Not used  MCA=Not used  MAXTEMP=Not used  CFGAN14=Not used  CFGAN15=Not used  S1IOL1WAY=Not used  S1BSSO=Not used  S1BACKBUG=Not used  BISTDIS=mBIST on reset feature disabled  NOBTSWP=BOOTSWP instruction is disabled  S1BISTDIS=Secondary BIST on reset feature disabled  S1DMTIVTL=Not used  S1DMTIVTH=Not used  S1DMTCNTL=Not used  S1DMTCNTH=Not used  S1DMTDIS=Secondary Dead Man Timer is Disabled and can be enabled by software  BSEQ=Not used  IBSEQ=Not used  SMB3EN=SMBus 3.0 input levels  FUSBIDIO2=USBID pin is controlled by the USB2 module  FVBUSIO2=VBUSON pin is controlled by the USB2 module  FUSBIDIO1=USBID pin is controlled by the USB1 module  FVBUSIO1=VBUSON pin is controlled by the USB1 module  VBATBOREN=Enable ZPBOR during VBAT Mode  FDSEN=Enable DSEN bit in DSCON  BORSEL=BOR trip voltage 2.1v (Non-OPAMP deviced operation)  POSCFGAIN=Gain is G3  POSCAGCDLY=Settling time = 25ms x AGCRNG  POSCAGCRNG=Range 1x  POSCAGC=Automatic Gain Control for Oscillator  FDBGWP=Not used  FDEVOPT_ODPUR0=OD pull-up Resistance disabled  FDEVOPT_ODPUR1=OD pull-up Resistance disabled  FDEVOPT_ODPUR2=OD pull-up Resistance disabled  FDEVOPT_ODPUR3=OD pull-up Resistance disabled
      settings: SourceProductName=MPLAB Device Blocks for Simulink
  Mux : Mux  Inputs=2
  Mux1 : Mux  Inputs=2
  Op-Amp : MCHP_Blockset/Analog IO/Op-Amp  Priority=-2000  OpAmp1=Enabled with positive and negative inputs  OpAmp2=Enabled with positive and negative inputs  OpAmp3=Enabled with positive and negative inputs  S_INPUT=[-1]  S_INPUT_Size=[3]  S_OUTPUT=[]  S_OUTPUT_Size=[]  S_ListCustomDatatype=S.S_ListCustomDatatype={};  MCHP_USER_INTERRUPTS=0  MCHP_PORT={OA1 Output}{OA1out}14:2:A2;{OA1 IN+}{OA1in+}14:2:A4;{OA1 IN-}{OA1in-}14:2:A3;{OA2 Output}{OA2out}14:2:B0;{OA2 IN+}{OA2in+}14:2:B2;{OA2 IN-}{OA2in-}14:2:B1;{OA3 Output}{OA3out}14:2:A5;{OA3 IN+}{OA3in+}14:2:B5;{OA3 IN-}{OA3in-}14:2:A6;  MCHP_MASTERLINK=Lab3_HallLog_hw_solution/BOARD MCLV-48V-300W dsPIC33AK512MC510 MC DIM1/Microchip Master  MCHP_CRC=622109
      settings: SourceProductName=MPLAB Device Blocks for Simulink
  PWM_HS_FEP : MCHP_Blockset/PWM IO/PWM_HS_FEP  Priority=-2000  PWM_APWM_Select=PWM (main)  PWMx_MODSEL=Center Aligned  PWMx_CLKSEL=no scaling  PWMx_TRGMOD=Free-running (continuous)  PWMx_TRGCNT=1  PWM_ClockResolution_DIVSEL_TXT=auto  PWM_ClockResolution_FSCL_TXT="Resol: 0.275(us)  -  MaxPer: 0.018(s)"  PWM_ClockResolution_NoScaling_TXT=Dynamic Options  MaxPeriod_s=50e-6  InitPeriode_s=50e-6  InitDutyCycleP_s=25e-6  InitDutyCycleS_s=10e-6  InitPhase_s=-1  InitPhaseL_s=0  evalin_ws=PWM1max=MCHP_Fun.Hex2num('40B3880000000000');PWM2max=MCHP_Fun.Hex2num('40B3880000000000');PWM3max=MCHP_Fun.Hex2num('40B3880000000000');  SampleTime=-1  S_INPUT=[-1]  S_INPUT_Size=[3]  S_OUTPUT=[]  S_OUTPUT_Size=[]  S_ListCustomDatatype=S.S_ListCustomDatatype={};  MCHP_USER_INTERRUPTS={PWM1}{PWM Generator 1}{PWM Generator 1 Interrupt}{VectorName(PWM1Interrupt) Priority(-1) };{PWM2}{PWM Generator 2}{PWM Generator 2 Interrupt}{VectorName(PWM2Interrupt) Priority(-1) };{PWM3}{PWM Generator 3}{PWM Generator 3 Interrupt}{VectorName(PWM3Interrupt) Priority(-1) };  MCHP_PORT={PWM1H}{PWM1H}32:1:P51;{PWM2H}{PWM2H}32:1:P49;{PWM3H}{PWM3H}32:1:P36;{PWM1L}{PWM1L}32:1:P52;{PWM2L}{PWM2L}32:1:P50;{PWM3L}{PWM3L}32:1:P37;  MCHP_MASTERLINK=Lab3_HallLog_hw_solution/BOARD MCLV-48V-300W dsPIC33AK512MC510 MC DIM1/Microchip Master  MCHP_CRC=7204052  PWMx_PMOD=Complementary  PWM1_HL=PWMxH & PWMxL output enabled  PWM1_H_PPS_TXT=D2 / P51 / Pin[82]  PWM1_L_PPS_TXT=D3 / P52 / Pin[83]  PWM1_swap=off  PWM1H_pol=off  PWM1L_pol=off  PWM2_HL=PWMxH & PWMxL output enabled  PWM2_H_PPS_TXT=D0 / P49 / Pin[78]  PWM2_L_PPS_TXT=D1 / P50 / Pin[79]  PWM2_swap=off  PWM2H_pol=off  PWM2L_pol=off  PWM3_HL=PWMxH & PWMxL output enabled  PWM3_H_PPS_TXT=C3 / P36 / Pin[66]  PWM3_L_PPS_TXT=C4 / P37 / Pin[67]  PWM3_swap=off  PWM3H_pol=off  PWM3L_pol=off  PWM4_HL=not used  PWM4_H_PPS_TXT=C2 / P35 / Pin[64]  PWM4_L_PPS_TXT=C5 / P38 / Pin[65]  PWM4_swap=off  PWM4H_pol=off  PWM4L_pol=off  PWM5_HL=not used  PWM5_H_PPS_TXT=D5 / P54 / Pin[90]  PWM5_L_PPS_TXT=D6 / P55 / Pin[91]  PWM5_swap=off  PWM5H_pol=off  PWM5L_pol=off  PWM6_HL=not used  PWM6_H_PPS_TXT=D9 / P58 / Pin[76]  PWM6_L_PPS_TXT=D10 / P59 / Pin[77]  PWM6_swap=off  PWM6H_pol=off  PWM6L_pol=off  PWM7_HL=not used  PWM7_H_PPS_TXT=C10 / P43 / Pin[68]  PWM7_L_PPS_TXT=C11 / P44 / Pin[69]  PWM7_swap=off  PWM7H_pol=off  PWM7L_pol=off  PWM8_HL=not used  PWM8_H_PPS_TXT=C12 / P45 / Pin[70]  PWM9_H_PPS_TXT=Dynamic Options  PWM10_H_PPS_TXT=Dynamic Options  PWM11_H_PPS_TXT=Dynamic Options  PWM12_H_PPS_TXT=Dynamic Options  PWM8_L_PPS_TXT=C13 / P46 / Pin[71]  PWM9_L_PPS_TXT=Dynamic Options  PWM10_L_PPS_TXT=Dynamic Options  PWM11_L_PPS_TXT=Dynamic Options  PWM12_L_PPS_TXT=Dynamic Options  PWM8_swap=off  PWM8H_pol=off  PWM8L_pol=off  PWM9_HL=not used  PWM9_swap=off  PWM9H_pol=off  PWM9L_pol=off  PWM10_HL=not used  PWM10_swap=off  PWM10H_pol=off  PWM10L_pol=off  PWM11_HL=not used  PWM11_swap=off  PWM11H_pol=off  PWM11L_pol=off  PWM12_HL=not used  PWM12_swap=off  PWM12H_pol=off  PWM12L_pol=off  PWM1_ShowTrig=on  PWM1_Init_PGxTRIGABC_s=[0 -1 -1 ]  PWM1_ADTRxEN1=ADC Trigger 1  PWM1_ADTRxEN2=none  PWM1_ADTRxEN3=none  PWM2_ShowTrig=off  PWM2_Init_PGxTRIGABC_s=[-1 -1 -1]  PWM2_ADTRxEN1=none  PWM2_ADTRxEN2=none  PWM2_ADTRxEN3=none  PWM3_ShowTrig=off  PWM3_Init_PGxTRIGABC_s=[-1 -1 -1]  PWM3_ADTRxEN1=none  PWM3_ADTRxEN2=none  PWM3_ADTRxEN3=none  PWM4_ShowTrig=off  PWM4_Init_PGxTRIGABC_s=[-1 -1 -1]  PWM4_ADTRxEN1=none  PWM4_ADTRxEN2=none  PWM4_ADTRxEN3=none  PWM5_ShowTrig=off  PWM5_Init_PGxTRIGABC_s=[-1 -1 -1]  PWM5_ADTRxEN1=none  PWM5_ADTRxEN2=none  PWM5_ADTRxEN3=none  PWM6_ShowTrig=off  PWM6_Init_PGxTRIGABC_s=[-1 -1 -1]  PWM6_ADTRxEN1=none  PWM6_ADTRxEN2=none  PWM6_ADTRxEN3=none  PWM7_ShowTrig=off  PWM7_Init_PGxTRIGABC_s=[-1 -1 -1]  PWM7_ADTRxEN1=none  PWM7_ADTRxEN2=none  PWM7_ADTRxEN3=none  PWM8_ShowTrig=off  PWM9_ShowTrig=off  PWM10_ShowTrig=off  PWM11_ShowTrig=off  PWM12_ShowTrig=off  PWM8_Init_PGxTRIGABC_s=[-1 -1 -1]  PWM9_Init_PGxTRIGABC_s=[-1 -1 -1]  PWM10_Init_PGxTRIGABC_s=[-1 -1 -1]  PWM11_Init_PGxTRIGABC_s=[-1 -1 -1]  PWM12_Init_PGxTRIGABC_s=[-1 -1 -1]  PWM8_ADTRxEN1=none  PWM9_ADTRxEN1=none  PWM10_ADTRxEN1=none  PWM11_ADTRxEN1=none  PWM12_ADTRxEN1=none  PWM8_ADTRxEN2=none  PWM9_ADTRxEN2=none  PWM10_ADTRxEN2=none  PWM11_ADTRxEN2=none  PWM12_ADTRxEN2=none  PWM8_ADTRxEN3=none  PWM9_ADTRxEN3=none  PWM10_ADTRxEN3=none  PWM11_ADTRxEN3=none  PWM12_ADTRxEN3=none  BlockInput_VectorScalar=Vectors (grouped by function)  BlockInput_Period=Not a block input  BlockInput_DutyCycle=a Floating Point input within range [0 1]  BlockInput_PhaseShift=Not a block input  BlockInput_PhaseShift_L=Not a block input  BlockInput_SEVTCMP=Not a block input  BlockInput_TRIGx=Not a block input  BlockInput_DeadTime=Not a block input  BlockOutput_FaultDisabled=off  BlockOutput_Fault=on  DTC=Positive dead time (ensure period of time with PWM_H and PWM_L disasserted)  FLTSRC1_DTCMP_TXT=<empty>  FLTSRC2_DTCMP_TXT=<empty>  FLTSRC3_DTCMP_TXT=<empty>  FLTSRC4_DTCMP_TXT=<empty>  FLTSRC5_DTCMP_TXT=<empty>  FLTSRC6_DTCMP_TXT=<empty>  FLTSRC7_DTCMP_TXT=<empty>  FLTSRC8_DTCMP_TXT=<empty>  FLTSRC9_DTCMP_TXT=<empty>  FLTSRC10_DTCMP_TXT=<empty>  FLTSRC11_DTCMP_TXT=<empty>  FLTSRC12_DTCMP_TXT=<empty>  DeadTime_s=1e-6  DeadTimeAlt_s=1e-6  DeadTimeComp_s=0  FLTMODx=Disabled  FLTSRCx_TXT=<empty>  FLTDATx=PWM H/L -> 11  CLMODx=Disabled  CLSRCx_TXT=<empty>  CLDATx=PWM H/L -> 00  FLTLEBENx=off  CLLEBENx=off  LeadEdgeBlkPer_s=5e-7  PHRx=off  PHFx=off  PLRx=off  PLFx=off  PWM_EVTA_EN_TXT=Not Used  PWM_EVTA_Source=PG1  PWM_EVTA_Select=EOC (End of Cycle)  PWM_EVTA_POL=off  PWM_EVTA_STRD=off  PWM_EVTA_SYNC=off  PWM_EVTB_EN_TXT=Not Used  PWM_EVTB_Source=PG1  PWM_EVTB_Select=EOC (End of Cycle)  PWM_EVTB_POL=off  PWM_EVTB_STRD=off  PWM_EVTB_SYNC=off  PWM_EVTC_EN_TXT=Not Used  PWM_EVTC_Source=PG1  PWM_EVTC_Select=EOC (End of Cycle)  PWM_EVTC_POL=off  PWM_EVTC_STRD=off  PWM_EVTC_SYNC=off  PWM_EVTD_EN_TXT=Not Used  PWM_EVTD_Source=PG1  PWM_EVTD_Select=EOC (End of Cycle)  PWM_EVTD_POL=off  PWM_EVTD_STRD=off  PWM_EVTD_SYNC=off  PWM_EVTE_EN_TXT=Not connected  PWM_EVTE_Source=PG1  PWM_EVTE_Select=EOC (End of Cycle)  PWM_EVTE_POL=off  PWM_EVTE_STRD=off  PWM_EVTE_SYNC=off  PWM_EVTF_EN_TXT=Not connected  PWM_EVTF_Source=PG1  PWM_EVTF_Select=EOC (End of Cycle)  PWM_EVTF_POL=off  PWM_EVTF_STRD=off  PWM_EVTF_SYNC=off
      settings: SourceProductName=MPLAB Device Blocks for Simulink
  Port Info : MCHP_Blockset/System Info/Port Info  MCHP_MASTERLINK=Lab3_HallLog_hw_solution/BOARD MCLV-48V-300W dsPIC33AK512MC510 MC DIM1/Microchip Master
      settings: SourceProductName=MPLAB Device Blocks for Simulink
  QEI1 : MCHP_Blockset/QEI/QEI  QEI_REF=1  QEI_MODE=Quadrature Encoder  QEI_x2mode=off  QEI_PulseCountDir=Down  PIN_QEA_TXT=D14 / P63 / Pin[96]  PIN_QEB_TXT=D13 / P62 / Pin[95]  SWPAB=off  QEAPOL=off  QEBPOL=off  SampleTime=50e-6  PIN_CCMP_TXT=A4 / P20 / Pin[33]  MCHP_USER_INTERRUPTS={QEI1}{QEI1 Position Counter}{QEI1 Position Counter Compare}{VectorName(QEI1Interrupt) Priority(-1) Config_BitSet(QEI1STATbits.PCHEQIEN) };  MCHP_PORT={QEI1 A}{QEIA1}5:0:P63;{QEI1 B}{QEIB1}5:0:P62;  MCHP_MASTERLINK=Lab3_HallLog_hw_solution/BOARD MCLV-48V-300W dsPIC33AK512MC510 MC DIM1/Microchip Master  INDXxCNT_Output=is not an output  POSxCNT_Output=is a 16 bits signed block output  RESET_Input=on  PIMOD_mode=position is cyclique between user defined boundaries  PIMOD_modeB=Never reset position  PIMOD_reset=on next INDEX event  PIN_INDEX_TXT=D12 / P61 / Pin[94]  IMV=QEA = 0 and QEB = 0  IMV_x2=QEA = 1  PIN_HOME_TXT=B0 / P17 / Pin[31]  QEIxLEC_GEC=[0 (QEIResolution-1)]  QEIxIC=0  PCIIRQ=off  IDXPOL=on  HOMPOL=on  VELxCNT_Output=is a 16 bits signed block output  INTxHLD_Output=is not an output  MaxPeriod=1e-3  FILTREN=on  QFDIV_popup_TXT=520.83 kHz  FILTER_CutOffFreq=100e3  QEI_IntPri=5
      settings: SourceProductName=MPLAB Device Blocks for Simulink
  Rate Transition3 : RateTransition  Deterministic=off
  SW1 : MCHP_Blockset/Digital IO/Digital Input  PORT_TXT="A   [ 0 : 15 ]"  PIN=12  INPUT_PIN_MODE=Hi-impedance (default)  PACK=off  SIMULTANEOUS=off  ORDERING=None  SampleTime=-1  MCHP_PORT={Digital In}{DIN}2:0:A12;  MCHP_MASTERLINK=Lab3_HallLog_hw_solution/BOARD MCLV-48V-300W dsPIC33AK512MC510 MC DIM1/Microchip Master
      settings: SourceProductName=MPLAB Device Blocks for Simulink
  SW2 : MCHP_Blockset/Digital IO/Digital Input  PORT_TXT="E   [ 0 : 4 ]"  PIN=1  INPUT_PIN_MODE=Hi-impedance (default)  PACK=off  SIMULTANEOUS=off  ORDERING=None  SampleTime=-1  MCHP_PORT={Digital In}{DIN}2:0:E1;  MCHP_MASTERLINK=Lab3_HallLog_hw_solution/BOARD MCLV-48V-300W dsPIC33AK512MC510 MC DIM1/Microchip Master
      settings: SourceProductName=MPLAB Device Blocks for Simulink
  SinCos : Trigonometry  Operator=sincos  OutputSignalType=real  AngleUnit=revolution
  Temp offset : Bias  Bias=-50  SaturateOnIntegerOverflow=off
  Temperature Gain : Gain  Gain=(3.3/65536/0.010)  OutDataTypeStr=single
  Timer Info : MCHP_Blockset/System Info/Timer Info  MCHP_MASTERLINK=Lab3_HallLog_hw_solution/BOARD MCLV-48V-300W dsPIC33AK512MC510 MC DIM1/Microchip Master
      settings: SourceProductName=MPLAB Device Blocks for Simulink
  Timing Analysis : Subsystem
  UART Configuration DEBUG (USB) : MCHP_Blockset/BUS UART/UART Configuration  UART_REF=1  BAUD_Choice_TXT="460800         [+0.01%]"  BAUD_Choice_IR_TXT=[]  BAUD_Custom=115200  INT_PRIORITY=0  ALT_IO=on  PIN_RX_TXT=C14 / P47 / Pin[74]  PIN_RX_INPUT_MODE=Hi-impedance (default)  PIN_TX_TXT=C15 / P48 / Pin[75]  PIN_TX_OUTPUT_MODE=Push-Pull (default)  MCHP_USER_INTERRUPTS={DMA2}{DMA Channel 2 (UART1 TX)}{DMA Channel 2 (UART1 TX)}{VectorName(DMA2Interrupt) Priority(5) };{DMA4}{DMA Channel 4 (UART1 RX)}{DMA Channel 4 (UART1 RX buffer event - no register read)}{VectorName(DMA4Interrupt) Priority(-1) };  MCHP_PORT="{UART1  Rx}{U1RX}3:0:P47;{UART1  Tx}{U1TX}3:0:P48;"  MCHP_MASTERLINK=Lab3_HallLog_hw_solution/BOARD MCLV-48V-300W dsPIC33AK512MC510 MC DIM1/Microchip Master  MCHP_COM_ExtPil=on  TX_IMPLEMENTATION=DMA Circular Buffer  TX_IMPLEMENTATION_default=Circular Buffer  TX_INT_PRIORITY=5  TX_INT_WHEN=is empty & last char is sent  TX_INT_WHEN_default=is empty & last char is sent  TX_CIRCULAR_SIZE=64  TX_DMA_CHANNEL=2  TX_DMA_SIZE=16  TX_TASK_PROTECTION=Delay tasks (default)  TX_INTERRUPT_PROTECTION=Do not send on conflict (default)  TX_INTERRUPT_PROTECTION_default=Do not send on conflict (default)  RX_IMPLEMENTATION=DMA Circular Buffer  RX_IMPLEMENTATION_default=Circular Buffer  RX_INT_PRIORITY=6  RX_INT_WHEN=receive 1 character  RX_CIRCULAR_SIZE=64  RX_DMA_CHANNEL=4  RX_DMA_SIZE=0  DuplexMode=Full duplex (default)  PIN_RX_Inv=off  PIN_TX_Inv=off  PIN_RXTX_Inv=off  ParityBit=No parity (default)  StopBit=1 stop bit (default)  IRDA=off  IdleTime_choice_TXT=None  IdleTime_custom=2/50  FlowControl=None  PIN_CTS_TXT=B0 / P17 / Pin[31]  PIN_CTS_INPUT_MODE=Hi-impedance (default)  PIN_RTS_TXT=B0 / P17 / Pin[31]  PIN_RTS_OUTPUT_MODE=Push-Pull (default)  PIN_DSR_TXT=B0 / P17 / Pin[31]  PIN_DSR_INPUT_MODE=Hi-impedance (default)  PIN_DTR_TXT=B0 / P17 / Pin[31]  PIN_DTR_OUTPUT_MODE=Push-Pull (default)  InitSequence_chkbox=off  BAUD_Choice_InitSeq_TXT="110         [+73.40%]"  BAUD_Choice_IR_InitSeq_TXT=0  BAUD_Custom_InitSeq=0  InitSequence="uint8(['use VT100 terminal ! ' 13 10 27 'c'  27 '[2J' ] )"
      settings: SourceProductName=MPLAB Device Blocks for Simulink
  "UART Configuration J11 - XPRO 1 Rx  #13, Tx #14" : MCHP_Blockset/BUS UART/UART Configuration  Commented=on  UART_REF=2  BAUD_Choice_TXT="2000000         [+0.00%]"  BAUD_Choice_IR_TXT=[]  BAUD_Custom=115200  INT_PRIORITY=0  ALT_IO=on  PIN_RX_TXT=C11 / P44 / Pin[69]  PIN_RX_INPUT_MODE=Hi-impedance (default)  PIN_TX_TXT=C10 / P43 / Pin[68]  PIN_TX_OUTPUT_MODE=Push-Pull (default)  MCHP_USER_INTERRUPTS={U2RX}{UART2 RX}{UART2 Receive Data Ready}{VectorName(U2RXInterrupt) Priority(6) RegisterReadClear(U2RXREG)};{U2TX}{UART2 TX}{UART2 Transmit Buffer Empty}{VectorName(U2TXInterrupt) Priority(5) };{U2E}{UART2 Error}{UART2 Error/Event}{VectorName(U2EInterrupt) Priority(-1) BitfieldClear(U2STATbits.RXFOIF=1|Overflow) BitfieldClear(U2STATbits.FERIF=1|Framing) BitfieldClear(U2STATbits.PERIF=1|Parity) };  MCHP_PORT="{UART2  Rx}{U2RX}3:0:P44;{UART2  Tx}{U2TX}3:0:P43;"  MCHP_MASTERLINK=Lab3_HallLog_hw_solution/BOARD MCLV-48V-300W dsPIC33AK512MC510 MC DIM1/Microchip Master  MCHP_COM_ExtPil=off  TX_IMPLEMENTATION=Circular Buffer  TX_IMPLEMENTATION_default=Circular Buffer  TX_INT_PRIORITY=5  TX_INT_WHEN=is empty  TX_INT_WHEN_default=is empty & last char is sent  TX_CIRCULAR_SIZE=512  TX_DMA_CHANNEL=1  TX_DMA_SIZE=[]  TX_TASK_PROTECTION=Delay tasks (default)  TX_INTERRUPT_PROTECTION=Do not send on conflict (default)  TX_INTERRUPT_PROTECTION_default=Do not send on conflict (default)  RX_IMPLEMENTATION=Circular Buffer  RX_IMPLEMENTATION_default=Circular Buffer  RX_INT_PRIORITY=6  RX_INT_WHEN=is 3/4 fulll (contains 3 data characters)  RX_CIRCULAR_SIZE=256  RX_DMA_CHANNEL="0   (Lowest Priority)"  RX_DMA_SIZE=0  DuplexMode=Full duplex (default)  PIN_RX_Inv=off  PIN_TX_Inv=off  PIN_RXTX_Inv=off  ParityBit=No parity (default)  StopBit=1 stop bit (default)  IRDA=off  IdleTime_choice_TXT=None  IdleTime_custom=2/50  FlowControl=None  PIN_CTS_TXT=A0 / P1 / Pin[4]  PIN_CTS_INPUT_MODE=Hi-impedance (default)  PIN_RTS_TXT=A0 / P1 / Pin[4]  PIN_RTS_OUTPUT_MODE=Push-Pull (default)  PIN_DSR_TXT=A0 / P1 / Pin[4]  PIN_DSR_INPUT_MODE=Hi-impedance (default)  PIN_DTR_TXT=A0 / P1 / Pin[4]  PIN_DTR_OUTPUT_MODE=Push-Pull (default)  InitSequence_chkbox=off  BAUD_Choice_InitSeq_TXT="110         [+73.40%]"  BAUD_Choice_IR_InitSeq_TXT=0  BAUD_Custom_InitSeq=0  InitSequence='Hello World'
      settings: SourceProductName=MPLAB Device Blocks for Simulink
  Weighted Sample Time : SampleTimeMath  TsampMathOp=/  weightValue=QEIResolution / (2*pi)  OutDataTypeStr=Inherit: Inherit via back propagation
  electrical position : Gain  Gain=n/QEIResolution  OutDataTypeStr=fixdt(0,16,16)
  fract range: 0-21V : DataTypeConversion  OutDataTypeStr=fixdt(0,16,3.3/65536*21,0)  ConvertRealWorld=Stored Integer (SI)  SaturateOnIntegerOverflow=off  RndMeth=Floor
  mechanical position : Gain  Gain=1/QEIResolution  OutDataTypeStr=fixdt(0,16,16)
  per_unit : Subsystem
  range: +- 22.0441A : DataTypeConversion  OutDataTypeStr=fixdt(1,16,22.0441/32768,0)  ConvertRealWorld=Stored Integer (SI)  SaturateOnIntegerOverflow=off  RndMeth=Floor
  range: +- 22.0441_ : DataTypeConversion  OutDataTypeStr=fixdt(1,16,22.0441/32768,0)  ConvertRealWorld=Stored Integer (SI)  SaturateOnIntegerOverflow=off  RndMeth=Floor
  unitary : DataTypeConversion  OutDataTypeStr=fixdt(0,16,16)  ConvertRealWorld=Stored Integer (SI)  SaturateOnIntegerOverflow=off  RndMeth=Floor
  sensors : Outport
  wires:
  Mux/1 -> Data Type Conversion1/1
  Gain/1 -> SinCos/1
  SinCos/2 -> Mux/2
  SinCos/1 -> Mux/1
  Center & sign reversal1/1(Iab) -> range: +- 22.0441_/1, per_unit/3(I_bus)
  Cast1/1 -> PWM_HS_FEP/1
  Encoder Offset_/1 -> Data Type Conversion3/1, Bus Creator3/2  "theta_m_unit"
  Encoder Offset/1 -> Data Type Conversion2/1, Bus Creator6/2, Gain/1  "theta_e_unit"
  Data Type Conversion3/1 -> Bus Creator3/1  "theta_m_rad"
  Mux1/1 -> Center & sign reversal/1(I_ab)
  Rate Transition3/1 -> Center & sign reversal1/2(Bias Update), Center & sign reversal/2(Bias Update)
  Center & sign reversal/1(Iab) -> per_unit/2(I_ab), range: +- 22.0441A/1
  Downsample x20 _/1(Out1) -> per_unit/4(V_bus), fract range: 0-21V/1  "U1 CH2"
  unitary/1 -> per_unit/1(pot), Bus Creator1/3  "pot"
  range: +- 22.0441_/1 -> Bus Creator1/2  "I_bus"
  Bus Creator7/1 -> Bus Creator4/3  "RAW"
  Data Type Conversion2/1 -> Bus Creator6/1  "theta_e_rad"
  per_unit/1(ADC_unit) -> Bus Creator5/4  "ADC_unit"
  reset encoder/1 -> QEI1/1
  LED 1/1 -> LED_1/1
  Bus Creator6/1 -> Bus Creator4/1  "elec"
  Bus Creator3/1 -> Bus Creator4/2  "mecc"
  PWM ]0 1[/1 -> Cast1/1
  Bus Creator5/1 -> sensors/1
  ADC/2(Ib) -> Mux1/2  "U1 CH2"
  INIT/1 -> Cast/1
  Bus Creator1/1 -> Bus Creator5/3  "ADC"
  fract range: 0-21V/1 -> Bus Creator1/4  "V_bus"
  range: +- 22.0441A/1 -> Bus Creator1/1  "I_ab"
  QEI1/2 -> Weighted Sample Time/1, Bus Creator7/1, Data Type Duplicate/1  "omega_RAW"
  Timing Analysis/1(CPU Load) -> Bus Creator2/1  "load"
  Timing Analysis/2(CPU Overload) -> Bus Creator2/2  "overload"
  Weighted Sample Time/1 -> Downsample Averaged x20/1(In1), Data Type Duplicate/2
  electrical position/1 -> Encoder Offset/1
  SW1/1 -> Bus Creator/1  "BTN 1"
  Downsample Averaged x20/1(Out1) -> Bus Creator3/3  "omega_m_rad"
  Bus Creator/1 -> Bus Creator5/2  "BTN"
  Bus Creator4/1 -> Bus Creator5/6  "optical coder"
  ADC/1(Ia) -> Mux1/1  "U1 CH1"
  Bus Creator2/1 -> Bus Creator5/1  "MCU"
  Downsample x20/1(Out1) -> unitary/1  "U1 CH1"
  ADC/5(V_BUS) -> Downsample x20 _/1(In1)
  mechanical position/1 -> Encoder Offset_/1
  Data Type Conversion1/1 -> Bus Creator6/3  "SinCos_th"
  QEI1/1 -> electrical position/1, mechanical position/1, Bus Creator7/2  "theta_RAW"
  SW2/1 -> Bus Creator/2  "BTN 2"
  LED 2/1 -> LED_2/1
  Constant/1 -> Bus Creator/3  "BTN 3"
  ADC/4(pot) -> Downsample x20/1(In1)
  LED 3/1 -> LED_PIM/1
  Cast/1 -> Rate Transition3/1
  ADC/3(IBus) -> Center & sign reversal1/1(I_ab)
  ADC/6(TEMP FET) -> Downsample x20 _1/1(In1)
  Downsample x20 _1/1(Out1) -> Temperature Gain/1  "U1 CH2"
  Temperature Gain/1 -> Temp offset/1
  Temp offset/1 -> Bus Creator5/5  "Temp"
